simulink model "polymorphism"  (Simulink 7.7)
settings: Solver=FixedStepDiscrete  StartTime=0.0  StopTime=10.0  FixedStep=1  RelTol=1e-3
libraries: mylibrary x2
settings Model: Creator=hnine  LastModifiedBy=hnine

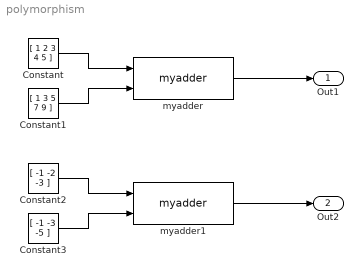
== system polymorphism ==
  Constant : Constant  Value=[ 1 2 3 4 5 ]
  Constant1 : Constant  Value=[ 1 3 5 7 9 ]
  Constant2 : Constant  Value=[ -1 -2 -3 ]
  Constant3 : Constant  Value=[ -1 -3 -5 ]
  myadder : mylibrary/myadder  SystemSampleTime=-1
  myadder1 : mylibrary/myadder  SystemSampleTime=-1
  Out1 : Outport
  Out2 : Outport  Port=2
  wires:
  Constant/1 -> myadder/1
  Constant1/1 -> myadder/2
  Constant2/1 -> myadder1/1
  Constant3/1 -> myadder1/2
  myadder/1 -> Out1/1
  myadder1/1 -> Out2/1
